simulink model "sine"  (R2020a)
settings: Solver=ode1  StartTime=0.0  StopTime=10.0  RelTol=1e-3
PostLoadFcn:
  | if any(exist('dsrtsu_mdlpostloadfcn', 'file') ~= 0), dsrtsu_mdlpostloadfcn('Execute', bdroot); end
InitFcn:
  | , if any(exist('rtifpga_mdlclblib', 'file') ~= 0), rtifpga_mdlclblib('Init', bdroot); end,
  | , if any(exist('dsmpb_private', 'file') ~= 0), dsmpb_private('dsmpb_mdlclblib', 'Init', bdroot); end,
libraries: dsmpblib x1
PreSaveFcn:
  | , if any(exist('dsmpb_private', 'file') ~= 0), dsmpb_private('dsmpb_mdlclblib', 'PreSave', bdroot); end,
CloseFcn:
  | , if any(exist('dsmpb_private', 'file') ~= 0), dsmpb_private('dsmpb_mdlclblib', 'Close', bdroot); end,
settings Model: DSMPB_ID_DATA={'7',struct('BlockId','d344c83c-69ae-4b89-b1f8-cfb9e53e87b0','SignalIds',{{'0b14571f-1a5e-4966-8cfd-fed4931a264e'}})}  RTICANMMDATA=struct('GeneralSetupData',struct('modelroot','D:\github\dspace-modelica-example\dSpaceExample','generalsettings',struct('filesettings',struct('destfolder',struct('Name','RTICANMM_FILES','Check',1),'buildfolder',struct('Name','.','Check',1),'AbsDestfolder',struct('Name','D:\github\dspace-modelica-example\dSpaceExample\RTICANMM_FILES'),'AbsBuildfolder',struct('Name','D:\github\dspace-modelica-example\dSpaceExample'))),'options',struct('addpaths',1,'rmpaths',1,'addtrcexclusion',true,'cannavigator',struct('checkmonitoring',0),'show_usrtrc',0,'use_usrtrc',0),'advanced',struct('options',ones(1,100)),'MPSetup',{{}},'RTI',struct('Type','GRT','Ver','','Date',''),'modelname','sine','block','sine'))  DSRTSU_INTERNAL_RTIFPGA=160  Creator=yangyang.fu  LastModifiedBy=yangyang.fu

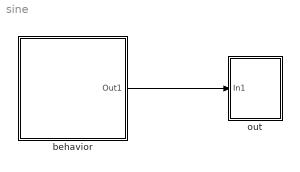
== system sine ==
  behavior : Subsystem
  out : Subsystem
  wires:
  behavior/1(Out1) -> out/1(In1)

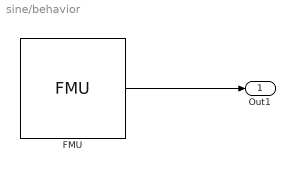
== system sine/behavior ==
  FMU : FMU  FMUName=testSine.fmu  FMUMode=CoSimulation  FMUSampleTime=0.01  sine=struct('amplitude',1,'freqHz',1,'phase',0,'offset',0,'startTime',0)  mask(testSine [Co-Simulation, v2.0]){}
      mask Display:
      | disp('testSine');
      | port_label('output',1,'y');
  Out1 : Outport
  wires:
  FMU/1 -> Out1/1

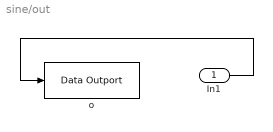
== system sine/out ==
  In1 : Inport
  o : dsmpblib/Data Outport  Priority=-10000
      settings: SourceProductName=dSPACE Model Interface Blockset
  wires:
  In1/1 -> o/1
